simulink model "sim12ex6"  (Simulink 2.09)
settings: Solver=ode45  StartTime=0.0  StopTime=20  MaxStep=.10  RelTol=1e-3  AbsTol=1e-3
settings Model: SaveTime=off  SaveOutput=off  ConsistencyChecking=off  RTWTemplateMakefile=grt_vc.tmf

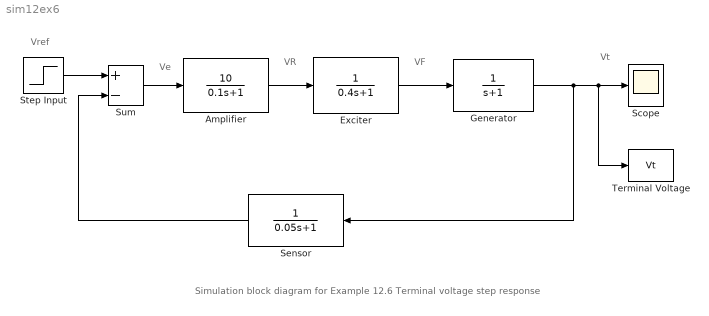
== system sim12ex6 ==
  note: Simulation block diagram for Example 12.6
      | Terminal voltage step response
  note: Vt
  note: VF
  note: VR
  note: Ve
  note: Vref
  Amplifier : TransferFcn  Numerator=[10]  Denominator="[0.1  1]"
  Exciter : TransferFcn  Numerator=[1]  Denominator="[0.4  1]"
  Generator : TransferFcn  Numerator=[1]  Denominator="[1  1]"
  Scope : Scope
      settings: TickLabels=on  TimeRange=auto  YMin=-5  YMax=5  SaveToWorkspace=off  SaveName=ScopeData
  Sensor : TransferFcn  Orientation=left  Numerator=[1]  Denominator="[0.05  1]"
  Step Input : Step  Time=20  Before=1  After=1
  Sum : Sum  Inputs=+-
  Terminal Voltage : ToWorkspace  VariableName=Vt  SampleTime=0
      settings: Buffer=1000
  wires:
  Generator/1 -> Terminal Voltage/1, Scope/1, Sensor/1
  Sensor/1 -> Sum/2
  Exciter/1 -> Generator/1
  Amplifier/1 -> Exciter/1
  Sum/1 -> Amplifier/1
  Step Input/1 -> Sum/1
